simulink model "disturbance-rejection"  (R2025b)
settings: Solver=VariableStepAuto  StartTime=0.0  StopTime=600  RelTol=1e-3
libraries: fuzblock x1
settings Model: Creator=kicam  LastModifiedBy=kicam

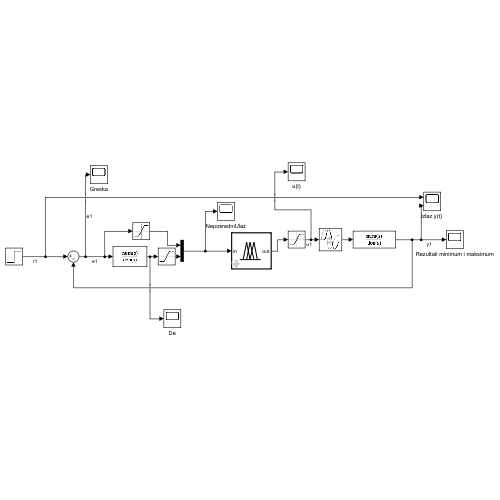
[thumbnail: Simulink's stored preview of the top-level diagram]
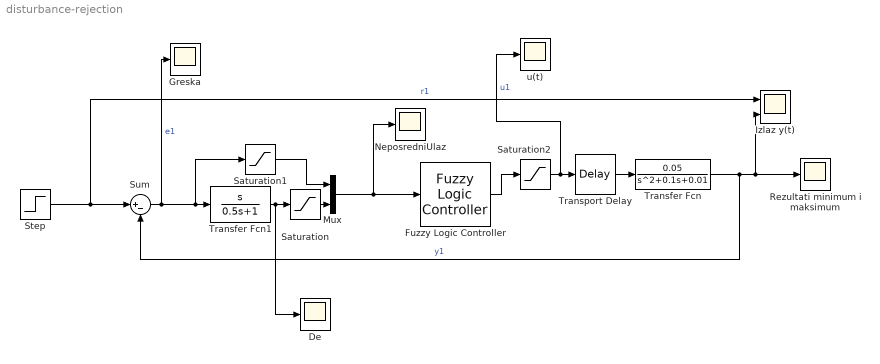
== system disturbance-rejection ==
  De : Scope
      settings: ActiveDisplayYMinimum=-1  ActiveDisplayYMaximum=1  DataLoggingVariableName=ScopeData4
  Fuzzy Logic Controller : fuzblock/Fuzzy Logic  Controller  FIS='mamdanitype1.fis'  OutputSampleNumber=101  DataType=double  UseLookupTable=off  NumBreakpoints=10  FuzzifiedInputs=off  RuleFiringStrengths=off  RuleOutputs=off  AggregatedOutputs=off  SimulateUsing=Interpreted execution  OutOfRangeInputValueMessage=warning  NoRuleFiredMessage=warning  EmptyOutputFuzzySetMessage=warning
  Greska : Scope
      settings: ActiveDisplayYMinimum=-1  ActiveDisplayYMaximum=1  DataLoggingVariableName=ScopeData3
  "Izlaz y(t) " : Scope  NumInputPorts=2
      settings: ActiveDisplayYMinimum=-25  ActiveDisplayYMaximum=25  DataLoggingVariableName=ScopeData2
  Mux : Mux  Inputs=2
  NeposredniUlaz : Scope
      settings: ActiveDisplayYMinimum=-26.765725460917352  ActiveDisplayYMaximum=40.891529148256183  DataLoggingVariableName=ScopeData5
  Rezultati minimum i maksimum : Scope
      settings: ActiveDisplayYMinimum=-18.227813441891492  ActiveDisplayYMaximum=22.792284103635104
  Saturation : Saturate  UpperLimit=20  LowerLimit=-20
  Saturation1 : Saturate  UpperLimit=50  LowerLimit=-50
  Saturation2 : Saturate  UpperLimit=10  LowerLimit=-10
  Step : Step  Time=20  Before=-20  After=20  SampleTime=0
  Sum : Sum  Inputs=|+-
  Transfer Fcn : TransferFcn  Numerator=[0.05]  Denominator=[1 0.1 0.01]
  Transfer Fcn1 : TransferFcn  Numerator=[1 0]  Denominator=[0.5 1]
  Transport Delay : TransportDelay  DelayTime=2
  u(t) : Scope
      settings: ActiveDisplayYMinimum=-1  ActiveDisplayYMaximum=1
  wires:
  Mux/1 -> NeposredniUlaz/1, Fuzzy Logic Controller/1
  Sum/1 -> Greska/1, Saturation1/1, Transfer Fcn1/1  "e1"
  Step/1 -> "Izlaz y(t) "/1, Sum/1  "r1"
  Transfer Fcn/1 -> "Izlaz y(t) "/2, Rezultati minimum i maksimum/1, Sum/2  "y1"
  Transport Delay/1 -> Transfer Fcn/1
  Saturation2/1 -> u(t)/1, Transport Delay/1  "u1"
  Transfer Fcn1/1 -> De/1, Saturation/1
  Saturation/1 -> Mux/2
  Fuzzy Logic Controller/1 -> Saturation2/1
  Saturation1/1 -> Mux/1
